simulink model "DynamicsAaa"  (R2017a)
(part 4 of 8)

v31 = 0.00359211102*c4*(- qd(3)*s3*(qd(1) + qd(2))) - 90*c4*(m6*(-c5*(- 295*c3^2*(qd(1) + qd(2))^2 + s2*(- 270*qd(1)^2) - 295*s3^2*(qd(1) + qd(2))^2) - s5*(c4*(+ c3*(c2*(- 270*qd(1)^2) - (qd(1) + qd(2))*(90*qd(1) + 90*qd(2)))) - s4*(- s3*(c2*(- 270*qd(1)^2) - (qd(1) + qd(2))*(90*qd(1) + 90*qd(2)))))) + m7*(c4*( - s3*(c2*(- 270*qd(1)^2) - (qd(1) + qd(2))*(90*qd(1) + 90*qd(2)))) + s4*( c3*(c2*(- 270*qd(1)^2) - (qd(1) + qd(2))*(90*qd(1) + 90*qd(2)))) + (-c5*(-qd(3) + qd(4)) - s5*(-c3*s4*(qd(1) + qd(2)) + c4*s3*(qd(1) + qd(2))))*(80*c5*(-qd(3) + qd(4)) + 80*s5*(-c3*s4*(qd(1) + qd(2)) + c4*s3*(qd(1) + qd(2)))) - (c5*(-c3*s4*(qd(1) + qd(2)) + c4*s3*(qd(1) + qd(2))) - s5*(-qd(3) + qd(4)))*(80*c5*(-c3*s4*(qd(1) + qd(2)) + c4*s3*(qd(1) + qd(2))) - 80*s5*(-qd(3) + qd(4))) - (-c6*(-c5*(-qd(3) + qd(4)) - s5*(-c3*s4*(qd(1) + qd(2)) + c4*s3*(qd(1) + qd(2)))) - s6*(c5*(-c3*s4*(qd(1) + qd(2)) + c4*s3*(qd(1) + qd(2))) - s5*(-qd(3) + qd(4))))*(80*c6*(-c5*(-qd(3) + qd(4)) - s5*(-c3*s4*(qd(1) + qd(2)) + c4*s3*(qd(1) + qd(2)))) + 80*s6*(c5*(-c3*s4*(qd(1) + qd(2)) + c4*s3*(qd(1) + qd(2))) - s5*(-qd(3) + qd(4)))) + (c6*(c5*(-c3*s4*(qd(1) + qd(2)) + c4*s3*(qd(1) + qd(2))) - s5*(-qd(3) + qd(4))) - s6*(-c5*(-qd(3) + qd(4)) - s5*(-c3*s4*(qd(1) + qd(2)) + c4*s3*(qd(1) + qd(2)))))*(80*c6*(c5*(-c3*s4*(qd(1) + qd(2)) + c4*s3*(qd(1) + qd(2))) - s5*(-qd(3) + qd(4))) - 80*s6*(-c5*(-qd(3) + qd(4)) - s5*(-c3*s4*(qd(1) + qd(2)) + c4*s3*(qd(1) + qd(2))))))) - 8.41256e-6*c4*(c3*qd(3)*(qd(1) + qd(2))) + c5*(-3.01352e-6*c6*(- qd(5)*(c5*(-c3*s4*(qd(1) + qd(2)) + c4*s3*(qd(1) + qd(2))) - s5*(-qd(3) + qd(4))) - s5*(c4*(c3*qd(3)*(qd(1) + qd(2))) + qd(4)*(-c3*c4*(qd(1) + qd(2)) - s3*s4*(qd(1) + qd(2))) - s4*( - qd(3)*s3*(qd(1) + qd(2))))) - 3.01352e-6*qd(6)*(c6*(c5*(-c3*s4*(qd(1) + qd(2)) + c4*s3*(qd(1) + qd(2))) - s5*(-qd(3) + qd(4))) - s6*(-c5*(-qd(3) + qd(4)) - s5*(-c3*s4*(qd(1) + qd(2)) + c4*s3*(qd(1) + qd(2))))) - 3.01352e-6*s6*(c5*(c4*(c3*qd(3)*(qd(1) + qd(2))) + qd(4)*(-c3*c4*(qd(1) + qd(2)) - s3*s4*(qd(1) + qd(2))) - s4*(- qd(3)*s3*(qd(1) + qd(2)))) + qd(5)*(-c5*(-qd(3) + qd(4)) - s5*(-c3*s4*(qd(1) + qd(2)) + c4*s3*(qd(1) + qd(2))))) + (6.20477e-6*c6*(c5*(-c3*s4*(qd(1) + qd(2)) + c4*s3*(qd(1) + qd(2))) - s5*(-qd(3) + qd(4))) - 6.20477e-6*s6*(-c5*(-qd(3) + qd(4)) - s5*(-c3*s4*(qd(1) + qd(2)) + c4*s3*(qd(1) + qd(2)))))*(c3*c4*(qd(1) + qd(2)) - qd(5) + qd(6) + s3*s4*(qd(1) + qd(2))) - (c6*(c5*(-c3*s4*(qd(1) + qd(2)) + c4*s3*(qd(1) + qd(2))) - s5*(-qd(3) + qd(4))) - s6*(-c5*(-qd(3) + qd(4)) - s5*(-c3*s4*(qd(1) + qd(2)) + c4*s3*(qd(1) + qd(2)))))*(3.29301e-6*c3*c4*(qd(1) + qd(2)) - 3.29301e-6*qd(5) + 3.29301e-6*qd(6) + 3.29301e-6*s3*s4*(qd(1) + qd(2)))) + 90*m5*(-c4*( - s3*(c2*(- 270*qd(1)^2) - (qd(1) + qd(2))*(90*qd(1) + 90*qd(2)))) + 295*c4*(c3*qd(3)*(qd(1) + qd(2))) + 295*qd(4)*(-c3*c4*(qd(1) + qd(2)) - s3*s4*(qd(1) + qd(2))) - s4*( c3*(c2*(- 270*qd(1)^2) - (qd(1) + qd(2))*(90*qd(1) + 90*qd(2)))) - 295*s4*(- qd(3)*s3*(qd(1) + qd(2))) + (-qd(3) + qd(4))*(295*c3*c4*(qd(1) + qd(2)) + 295*s3*s4*(qd(1) + qd(2)))) - 8.41256e-6*qd(4)*(-c3*c4*(qd(1) + qd(2)) - s3*s4*(qd(1) + qd(2))) + 0.00359211102*qd(4)*(-c3*s4*(qd(1) + qd(2)) + c4*s3*(qd(1) + qd(2))) + 8.41256e-6*s4*(- qd(3)*s3*(qd(1) + qd(2))) + 0.00359211102*s4*(c3*qd(3)*(qd(1) + qd(2))) - 90*s4*(c5*m7*(80*c6*(- qd(5)*(c5*(-c3*s4*(qd(1) + qd(2)) + c4*s3*(qd(1) + qd(2))) - s5*(-qd(3) + qd(4))) - s5*(c4*(c3*qd(3)*(qd(1) + qd(2))) + qd(4)*(-c3*c4*(qd(1) + qd(2)) - s3*s4*(qd(1) + qd(2))) - s4*(- qd(3)*s3*(qd(1) + qd(2))))) + c6*(c5*(c4*(c3*(c2*(- 270*qd(1)^2) - (qd(1) + qd(2))*(90*qd(1) + 90*qd(2)))) - s4*(- s3*(c2*(- 270*qd(1)^2) - (qd(1) + qd(2))*(90*qd(1) + 90*qd(2))))) + 80*qd(5)*(c5*(-c3*s4*(qd(1) + qd(2)) + c4*s3*(qd(1) + qd(2))) - s5*(-qd(3) + qd(4))) + 80*s5*(c4*(c3*qd(3)*(qd(1) + qd(2))) + qd(4)*(-c3*c4*(qd(1) + qd(2)) - s3*s4*(qd(1) + qd(2))) - s4*(- qd(3)*s3*(qd(1) + qd(2)))) - s5*(- 295*c3^2*(qd(1) + qd(2))^2 + s2*(- 270*qd(1)^2) - 295*s3^2*(qd(1) + qd(2))^2) - (80*c5*(-c3*s4*(qd(1) + qd(2)) + c4*s3*(qd(1) + qd(2))) - 80*s5*(-qd(3) + qd(4)))*(-c3*c4*(qd(1) + qd(2)) + qd(5) - s3*s4*(qd(1) + qd(2)))) + 80*qd(6)*(c6*(c5*(-c3*s4*(qd(1) + qd(2)) + c4*s3*(qd(1) + qd(2))) - s5*(-qd(3) + qd(4))) - s6*(-c5*(-qd(3) + qd(4)) - s5*(-c3*s4*(qd(1) + qd(2)) + c4*s3*(qd(1) + qd(2))))) + 80*s6*(c5*(c4*(c3*qd(3)*(qd(1) + qd(2))) + qd(4)*(-c3*c4*(qd(1) + qd(2)) - s3*s4*(qd(1) + qd(2))) - s4*(- qd(3)*s3*(qd(1) + qd(2)))) + qd(5)*(-c5*(-qd(3) + qd(4)) - s5*(-c3*s4*(qd(1) + qd(2)) + c4*s3*(qd(1) + qd(2))))) - s6*(80*c5*(c4*(c3*qd(3)*(qd(1) + qd(2))) + qd(4)*(-c3*c4*(qd(1) + qd(2)) - s3*s4*(qd(1) + qd(2))) - s4*(- qd(3)*s3*(qd(1) + qd(2)))) - c5*(- 295*c3^2*(qd(1) + qd(2))^2 + s2*(- 270*qd(1)^2) - 295*s3^2*(qd(1) + qd(2))^2) + 80*qd(5)*(-c5*(-qd(3) + qd(4)) - s5*(-c3*s4*(qd(1) + qd(2)) + c4*s3*(qd(1) + qd(2)))) - s5*(c4*(c3*(c2*(- 270*qd(1)^2) - (qd(1) + qd(2))*(90*qd(1) + 90*qd(2)))) - s4*(- s3*(c2*(- 270*qd(1)^2) - (qd(1) + qd(2))*(90*qd(1) + 90*qd(2))))) + (80*c5*(-qd(3) + qd(4)) + 80*s5*(-c3*s4*(qd(1) + qd(2)) + c4*s3*(qd(1) + qd(2))))*(-c3*c4*(qd(1) + qd(2)) + qd(5) - s3*s4*(qd(1) + qd(2)))) - (80*c6*(c5*(-c3*s4*(qd(1) + qd(2)) + c4*s3*(qd(1) + qd(2))) - s5*(-qd(3) + qd(4))) - 80*s6*(-c5*(-qd(3) + qd(4)) - s5*(-c3*s4*(qd(1) + qd(2)) + c4*s3*(qd(1) + qd(2)))))*(c3*c4*(qd(1) + qd(2)) - qd(5) + qd(6) + s3*s4*(qd(1) + qd(2)))) + m6*(c5*(c4*(c3*(c2*(- 270*qd(1)^2) - (qd(1) + qd(2))*(90*qd(1) + 90*qd(2)))) - s4*(- s3*(c2*(- 270*qd(1)^2) - (qd(1) + qd(2))*(90*qd(1) + 90*qd(2))))) - s5*( - 295*c3^2*(qd(1) + qd(2))^2 + s2*(- 270*qd(1)^2) - 295*s3^2*(qd(1) + qd(2))^2)) - m7*s5*(80*c6*(c5*(c4*(c3*qd(3)*(qd(1) + qd(2))) + qd(4)*(-c3*c4*(qd(1) + qd(2)) - s3*s4*(qd(1) + qd(2))) - s4*(- qd(3)*s3*(qd(1) + qd(2)))) + qd(5)*(-c5*(-qd(3) + qd(4)) - s5*(-c3*s4*(qd(1) + qd(2)) + c4*s3*(qd(1) + qd(2))))) - c6*(80*c5*(c4*(c3*qd(3)*(qd(1) + qd(2))) + qd(4)*(-c3*c4*(qd(1) + qd(2)) - s3*s4*(qd(1) + qd(2))) - s4*( - qd(3)*s3*(qd(1) + qd(2)))) - c5*( - 295*c3^2*(qd(1) + qd(2))^2 + s2*(- 270*qd(1)^2) - 295*s3^2*(qd(1) + qd(2))^2) + 80*qd(5)*(-c5*(-qd(3) + qd(4)) - s5*(-c3*s4*(qd(1) + qd(2)) + c4*s3*(qd(1) + qd(2)))) - s5*(c4*(c3*(c2*(- 270*qd(1)^2) - (qd(1) + qd(2))*(90*qd(1) + 90*qd(2)))) - s4*(- s3*(c2*(- 270*qd(1)^2) - (qd(1) + qd(2))*(90*qd(1) + 90*qd(2))))) + (80*c5*(-qd(3) + qd(4)) + 80*s5*(-c3*s4*(qd(1) + qd(2)) + c4*s3*(qd(1) + qd(2))))*(-c3*c4*(qd(1) + qd(2)) + qd(5) - s3*s4*(qd(1) + qd(2)))) + 80*qd(6)*(-c6*(-c5*(-qd(3) + qd(4)) - s5*(-c3*s4*(qd(1) + qd(2)) + c4*s3*(qd(1) + qd(2)))) - s6*(c5*(-c3*s4*(qd(1) + qd(2)) + c4*s3*(qd(1) + qd(2))) - s5*(-qd(3) + qd(4)))) - 80*s6*(- qd(5)*(c5*(-c3*s4*(qd(1) + qd(2)) + c4*s3*(qd(1) + qd(2))) - s5*(-qd(3) + qd(4))) - s5*(c4*(c3*qd(3)*(qd(1) + qd(2))) + qd(4)*(-c3*c4*(qd(1) + qd(2)) - s3*s4*(qd(1) + qd(2))) - s4*(- qd(3)*s3*(qd(1) + qd(2))))) - s6*(c5*(c4*(c3*(c2*(- 270*qd(1)^2) - (qd(1) + qd(2))*(90*qd(1) + 90*qd(2)))) - s4*( - s3*(c2*(- 270*qd(1)^2) - (qd(1) + qd(2))*(90*qd(1) + 90*qd(2))))) + 80*qd(5)*(c5*(-c3*s4*(qd(1) + qd(2)) + c4*s3*(qd(1) + qd(2))) - s5*(-qd(3) + qd(4))) + 80*s5*(c4*(c3*qd(3)*(qd(1) + qd(2))) + qd(4)*(-c3*c4*(qd(1) + qd(2)) - s3*s4*(qd(1) + qd(2))) - s4*(- qd(3)*s3*(qd(1) + qd(2)))) - s5*(- 295*c3^2*(qd(1) + qd(2))^2 + s2*(- 270*qd(1)^2) - 295*s3^2*(qd(1) + qd(2))^2) - (80*c5*(-c3*s4*(qd(1) + qd(2)) + c4*s3*(qd(1) + qd(2))) - 80*s5*(-qd(3) + qd(4)))*(-c3*c4*(qd(1) + qd(2)) + qd(5) - s3*s4*(qd(1) + qd(2)))) + (80*c6*(-c5*(-qd(3) + qd(4)) - s5*(-c3*s4*(qd(1) + qd(2)) + c4*s3*(qd(1) + qd(2)))) + 80*s6*(c5*(-c3*s4*(qd(1) + qd(2)) + c4*s3*(qd(1) + qd(2))) - s5*(-qd(3) + qd(4))))*(c3*c4*(qd(1) + qd(2)) - qd(5) + qd(6) + s3*s4*(qd(1) + qd(2))))) + s5*(6.20477e-6*c6*(c5*(c4*(c3*qd(3)*(qd(1) + qd(2))) + qd(4)*(-c3*c4*(qd(1) + qd(2)) - s3*s4*(qd(1) + qd(2))) - s4*(- qd(3)*s3*(qd(1) + qd(2)))) + qd(5)*(-c5*(-qd(3) + qd(4)) - s5*(-c3*s4*(qd(1) + qd(2)) + c4*s3*(qd(1) + qd(2))))) + 6.20477e-6*qd(6)*(-c6*(-c5*(-qd(3) + qd(4)) - s5*(-c3*s4*(qd(1) + qd(2)) + c4*s3*(qd(1) + qd(2)))) - s6*(c5*(-c3*s4*(qd(1) + qd(2)) + c4*s3*(qd(1) + qd(2))) - s5*(-qd(3) + qd(4)))) - 6.20477e-6*s6*(- qd(5)*(c5*(-c3*s4*(qd(1) + qd(2)) + c4*s3*(qd(1) + qd(2))) - s5*(-qd(3) + qd(4))) - s5*(c4*(c3*qd(3)*(qd(1) + qd(2))) + qd(4)*(-c3*c4*(qd(1) + qd(2)) - s3*s4*(qd(1) + qd(2))) - s4*(- qd(3)*s3*(qd(1) + qd(2))))) + (-c6*(-c5*(-qd(3) + qd(4)) - s5*(-c3*s4*(qd(1) + qd(2)) + c4*s3*(qd(1) + qd(2)))) - s6*(c5*(-c3*s4*(qd(1) + qd(2)) + c4*s3*(qd(1) + qd(2))) - s5*(-qd(3) + qd(4))))*(3.29301e-6*c3*c4*(qd(1) + qd(2)) - 3.29301e-6*qd(5) + 3.29301e-6*qd(6) + 3.29301e-6*s3*s4*(qd(1) + qd(2))) - (-3.01352e-6*c6*(-c5*(-qd(3) + qd(4)) - s5*(-c3*s4*(qd(1) + qd(2)) + c4*s3*(qd(1) + qd(2)))) - 3.01352e-6*s6*(c5*(-c3*s4*(qd(1) + qd(2)) + c4*s3*(qd(1) + qd(2))) - s5*(-qd(3) + qd(4))))*(c3*c4*(qd(1) + qd(2)) - qd(5) + qd(6) + s3*s4*(qd(1) + qd(2)))) + (-c5*(-qd(3) + qd(4)) - s5*(-c3*s4*(qd(1) + qd(2)) + c4*s3*(qd(1) + qd(2))))*(0.000409305*c5*(-qd(3) + qd(4)) + 0.00151607*c5*(-c3*s4*(qd(1) + qd(2)) + c4*s3*(qd(1) + qd(2))) - 0.00151607*s5*(-qd(3) + qd(4)) + 0.000409305*s5*(-c3*s4*(qd(1) + qd(2)) + c4*s3*(qd(1) + qd(2)))) - (c5*(-c3*s4*(qd(1) + qd(2)) + c4*s3*(qd(1) + qd(2))) - s5*(-qd(3) + qd(4)))*(-0.00355535*c5*(-qd(3) + qd(4)) - 0.000409305*c5*(-c3*s4*(qd(1) + qd(2)) + c4*s3*(qd(1) + qd(2))) + 0.000409305*s5*(-qd(3) + qd(4)) - 0.00355535*s5*(-c3*s4*(qd(1) + qd(2)) + c4*s3*(qd(1) + qd(2)))) - (-c3*c4*(qd(1) + qd(2)) - s3*s4*(qd(1) + qd(2)))*(0.00163355*c3*c4*(qd(1) + qd(2)) - 0.00950111*c3*s4*(qd(1) + qd(2)) + 0.00950111*c4*s3*(qd(1) + qd(2)) + 8.41256e-6*qd(3) - 8.41256e-6*qd(4) + 0.00163355*s3*s4*(qd(1) + qd(2))) + (-c3*s4*(qd(1) + qd(2)) + c4*s3*(qd(1) + qd(2)))*(-0.020170031*c3*c4*(qd(1) + qd(2)) + 0.00163355*c3*s4*(qd(1) + qd(2)) - 0.00163355*c4*s3*(qd(1) + qd(2)) + 2.69102e-6*qd(3) - 2.69102e-6*qd(4) - 0.020170031*s3*s4*(qd(1) + qd(2)));

v41 = -0.00358942*c4*( - qd(3)*s3*(qd(1) + qd(2))) - c5*(-3.01352e-6*c6*(- qd(5)*(c5*(-c3*s4*(qd(1) + qd(2)) + c4*s3*(qd(1) + qd(2))) - s5*(-qd(3) + qd(4))) - s5*(c4*(c3*qd(3)*(qd(1) + qd(2))) + qd(4)*(-c3*c4*(qd(1) + qd(2)) - s3*s4*(qd(1) + qd(2))) - s4*(- qd(3)*s3*(qd(1) + qd(2))))) - 3.01352e-6*qd(6)*(c6*(c5*(-c3*s4*(qd(1) + qd(2)) + c4*s3*(qd(1) + qd(2))) - s5*(-qd(3) + qd(4))) - s6*(-c5*(-qd(3) + qd(4)) - s5*(-c3*s4*(qd(1) + qd(2)) + c4*s3*(qd(1) + qd(2))))) - 3.01352e-6*s6*(c5*(c4*(c3*qd(3)*(qd(1) + qd(2))) + qd(4)*(-c3*c4*(qd(1) + qd(2)) - s3*s4*(qd(1) + qd(2))) - s4*(- qd(3)*s3*(qd(1) + qd(2)))) + qd(5)*(-c5*(-qd(3) + qd(4)) - s5*(-c3*s4*(qd(1) + qd(2)) + c4*s3*(qd(1) + qd(2))))) + (6.20477e-6*c6*(c5*(-c3*s4*(qd(1) + qd(2)) + c4*s3*(qd(1) + qd(2))) - s5*(-qd(3) + qd(4))) - 6.20477e-6*s6*(-c5*(-qd(3) + qd(4)) - s5*(-c3*s4*(qd(1) + qd(2)) + c4*s3*(qd(1) + qd(2)))))*(c3*c4*(qd(1) + qd(2)) - qd(5) + qd(6) + s3*s4*(qd(1) + qd(2))) - (c6*(c5*(-c3*s4*(qd(1) + qd(2)) + c4*s3*(qd(1) + qd(2))) - s5*(-qd(3) + qd(4))) - s6*(-c5*(-qd(3) + qd(4)) - s5*(-c3*s4*(qd(1) + qd(2)) + c4*s3*(qd(1) + qd(2)))))*(3.29301e-6*c3*c4*(qd(1) + qd(2)) - 3.29301e-6*qd(5) + 3.29301e-6*qd(6) + 3.29301e-6*s3*s4*(qd(1) + qd(2)))) - 0.00358942*qd(4)*(-c3*s4*(qd(1) + qd(2)) + c4*s3*(qd(1) + qd(2))) - 0.00358942*s4*(c3*qd(3)*(qd(1) + qd(2))) - s5*(6.20477e-6*c6*(c5*(c4*(c3*qd(3)*(qd(1) + qd(2))) + qd(4)*(-c3*c4*(qd(1) + qd(2)) - s3*s4*(qd(1) + qd(2))) - s4*( - qd(3)*s3*(qd(1) + qd(2)))) + qd(5)*(-c5*(-qd(3) + qd(4)) - s5*(-c3*s4*(qd(1) + qd(2)) + c4*s3*(qd(1) + qd(2))))) + 6.20477e-6*qd(6)*(-c6*(-c5*(-qd(3) + qd(4)) - s5*(-c3*s4*(qd(1) + qd(2)) + c4*s3*(qd(1) + qd(2)))) - s6*(c5*(-c3*s4*(qd(1) + qd(2)) + c4*s3*(qd(1) + qd(2))) - s5*(-qd(3) + qd(4)))) - 6.20477e-6*s6*(- qd(5)*(c5*(-c3*s4*(qd(1) + qd(2)) + c4*s3*(qd(1) + qd(2))) - s5*(-qd(3) + qd(4))) - s5*(c4*(c3*qd(3)*(qd(1) + qd(2))) + qd(4)*(-c3*c4*(qd(1) + qd(2)) - s3*s4*(qd(1) + qd(2))) - s4*(- qd(3)*s3*(qd(1) + qd(2))))) + (-c6*(-c5*(-qd(3) + qd(4)) - s5*(-c3*s4*(qd(1) + qd(2)) + c4*s3*(qd(1) + qd(2)))) - s6*(c5*(-c3*s4*(qd(1) + qd(2)) + c4*s3*(qd(1) + qd(2))) - s5*(-qd(3) + qd(4))))*(3.29301e-6*c3*c4*(qd(1) + qd(2)) - 3.29301e-6*qd(5) + 3.29301e-6*qd(6) + 3.29301e-6*s3*s4*(qd(1) + qd(2))) - (-3.01352e-6*c6*(-c5*(-qd(3) + qd(4)) - s5*(-c3*s4*(qd(1) + qd(2)) + c4*s3*(qd(1) + qd(2)))) - 3.01352e-6*s6*(c5*(-c3*s4*(qd(1) + qd(2)) + c4*s3*(qd(1) + qd(2))) - s5*(-qd(3) + qd(4))))*(c3*c4*(qd(1) + qd(2)) - qd(5) + qd(6) + s3*s4*(qd(1) + qd(2)))) - (-c5*(-qd(3) + qd(4)) - s5*(-c3*s4*(qd(1) + qd(2)) + c4*s3*(qd(1) + qd(2))))*(0.000409305*c5*(-qd(3) + qd(4)) + 0.00151607*c5*(-c3*s4*(qd(1) + qd(2)) + c4*s3*(qd(1) + qd(2))) - 0.00151607*s5*(-qd(3) + qd(4)) + 0.000409305*s5*(-c3*s4*(qd(1) + qd(2)) + c4*s3*(qd(1) + qd(2)))) + (c5*(-c3*s4*(qd(1) + qd(2)) + c4*s3*(qd(1) + qd(2))) - s5*(-qd(3) + qd(4)))*(-0.00355535*c5*(-qd(3) + qd(4)) - 0.000409305*c5*(-c3*s4*(qd(1) + qd(2)) + c4*s3*(qd(1) + qd(2))) + 0.000409305*s5*(-qd(3) + qd(4)) - 0.00355535*s5*(-c3*s4*(qd(1) + qd(2)) + c4*s3*(qd(1) + qd(2))));

v51 = 3.29301e-6*c4*(- qd(3)*s3*(qd(1) + qd(2))) + 3.29301e-6*qd(4)*(-c3*s4*(qd(1) + qd(2)) + c4*s3*(qd(1) + qd(2))) + 3.29301e-6*s4*(c3*qd(3)*(qd(1) + qd(2))) - (-c6*(-c5*(-qd(3) + qd(4)) - s5*(-c3*s4*(qd(1) + qd(2)) + c4*s3*(qd(1) + qd(2)))) - s6*(c5*(-c3*s4*(qd(1) + qd(2)) + c4*s3*(qd(1) + qd(2))) - s5*(-qd(3) + qd(4))))*(6.20477e-6*c6*(c5*(-c3*s4*(qd(1) + qd(2)) + c4*s3*(qd(1) + qd(2))) - s5*(-qd(3) + qd(4))) - 6.20477e-6*s6*(-c5*(-qd(3) + qd(4)) - s5*(-c3*s4*(qd(1) + qd(2)) + c4*s3*(qd(1) + qd(2))))) + (-3.01352e-6*c6*(-c5*(-qd(3) + qd(4)) - s5*(-c3*s4*(qd(1) + qd(2)) + c4*s3*(qd(1) + qd(2)))) - 3.01352e-6*s6*(c5*(-c3*s4*(qd(1) + qd(2)) + c4*s3*(qd(1) + qd(2))) - s5*(-qd(3) + qd(4))))*(c6*(c5*(-c3*s4*(qd(1) + qd(2)) + c4*s3*(qd(1) + qd(2))) - s5*(-qd(3) + qd(4))) - s6*(-c5*(-qd(3) + qd(4)) - s5*(-c3*s4*(qd(1) + qd(2)) + c4*s3*(qd(1) + qd(2)))));

v61 = 0;

V = [v11 ; v21 ; v31 ; v41 ; v51 ; v61];
%% matrix G



% g1 = diff(tau1,g)*g ;
% g2 = diff(tau2,g)*g ;
% g3 = diff(tau3,g)*g ;
% g4 = diff(tau4,g)*g ;
% g5 = diff(tau5,g)*g ;
% g6 = diff(tau6,g)*g ;

g1 = g*(335*c2*(c3*(m5*(s3*s4*(c1*s2 + c2*s1) + c3*c4*(c1*s2 + c2*s1)) - s4*(m7*(c3*s4*(c1*s2 + c2*s1) - c4*s3*(c1*s2 + c2*s1)) - m6*(s5*(s3*s4*(c1*s2 + c2*s1) + c3*c4*(c1*s2 + c2*s1)) - c5*(c1*c2 - s1*s2))) + c4*(m6*(c5*(s3*s4*(c1*s2 + c2*s1) + c3*c4*(c1*s2 + c2*s1)) + s5*(c1*c2 - s1*s2)) + c5*m7*(c6*(c5*(s3*s4*(c1*s2 + c2*s1) + c3*c4*(c1*s2 + c2*s1)) + s5*(c1*c2 - s1*s2)) + s6*(s5*(s3*s4*(c1*s2 + c2*s1) + c3*c4*(c1*s2 + c2*s1)) - c5*(c1*c2 - s1*s2))) - m7*s5*(c6*(s5*(s3*s4*(c1*s2 + c2*s1) + c3*c4*(c1*s2 + c2*s1)) - c5*(c1*c2 - s1*s2)) - s6*(c5*(s3*s4*(c1*s2 + c2*s1) + c3*c4*(c1*s2 + c2*s1)) + s5*(c1*c2 - s1*s2))))) + s3*(m5*(c3*s4*(c1*s2 + c2*s1) - c4*s3*(c1*s2 + c2*s1)) + c4*(m7*(c3*s4*(c1*s2 + c2*s1) - c4*s3*(c1*s2 + c2*s1)) - m6*(s5*(s3*s4*(c1*s2 + c2*s1) + c3*c4*(c1*s2 + c2*s1)) - c5*(c1*c2 - s1*s2))) + s4*(m6*(c5*(s3*s4*(c1*s2 + c2*s1) + c3*c4*(c1*s2 + c2*s1)) + s5*(c1*c2 - s1*s2)) + c5*m7*(c6*(c5*(s3*s4*(c1*s2 + c2*s1) + c3*c4*(c1*s2 + c2*s1)) + s5*(c1*c2 - s1*s2)) + s6*(s5*(s3*s4*(c1*s2 + c2*s1) + c3*c4*(c1*s2 + c2*s1)) - c5*(c1*c2 - s1*s2))) - m7*s5*(c6*(s5*(s3*s4*(c1*s2 + c2*s1) + c3*c4*(c1*s2 + c2*s1)) - c5*(c1*c2 - s1*s2)) - s6*(c5*(s3*s4*(c1*s2 + c2*s1) + c3*c4*(c1*s2 + c2*s1)) + s5*(c1*c2 - s1*s2))))) + c3*m4*(c1*s2 + c2*s1)) - 75*c2*(m6*(c3*s4*(c1*s2 + c2*s1) - c4*s3*(c1*s2 + c2*s1)) - m5*(c1*c2 - s1*s2) - m4*s3*(c1*s2 + c2*s1) + c5*m7*(c6*(s5*(s3*s4*(c1*s2 + c2*s1) + c3*c4*(c1*s2 + c2*s1)) - c5*(c1*c2 - s1*s2)) - s6*(c5*(s3*s4*(c1*s2 + c2*s1) + c3*c4*(c1*s2 + c2*s1)) + s5*(c1*c2 - s1*s2))) + m7*s5*(c6*(c5*(s3*s4*(c1*s2 + c2*s1) + c3*c4*(c1*s2 + c2*s1)) + s5*(c1*c2 - s1*s2)) + s6*(s5*(s3*s4*(c1*s2 + c2*s1) + c3*c4*(c1*s2 + c2*s1)) - c5*(c1*c2 - s1*s2)))) + c3*(90*m6*(c3*s4*(c1*s2 + c2*s1) - c4*s3*(c1*s2 + c2*s1)) + s4*(295*m7*(c3*s4*(c1*s2 + c2*s1) - c4*s3*(c1*s2 + c2*s1)) - 295*m6*(s5*(s3*s4*(c1*s2 + c2*s1) + c3*c4*(c1*s2 + c2*s1)) - c5*(c1*c2 - s1*s2))) - 90*m5*(c1*c2 - s1*s2) - c4*(295*m6*(c5*(s3*s4*(c1*s2 + c2*s1) + c3*c4*(c1*s2 + c2*s1)) + s5*(c1*c2 - s1*s2)) + 295*c5*m7*(c6*(c5*(s3*s4*(c1*s2 + c2*s1) + c3*c4*(c1*s2 + c2*s1)) + s5*(c1*c2 - s1*s2)) + s6*(s5*(s3*s4*(c1*s2 + c2*s1) + c3*c4*(c1*s2 + c2*s1)) - c5*(c1*c2 - s1*s2))) - 295*m7*s5*(c6*(s5*(s3*s4*(c1*s2 + c2*s1) + c3*c4*(c1*s2 + c2*s1)) - c5*(c1*c2 - s1*s2)) - s6*(c5*(s3*s4*(c1*s2 + c2*s1) + c3*c4*(c1*s2 + c2*s1)) + s5*(c1*c2 - s1*s2)))) + 90*c5*m7*(c6*(s5*(s3*s4*(c1*s2 + c2*s1) + c3*c4*(c1*s2 + c2*s1)) - c5*(c1*c2 - s1*s2)) - s6*(c5*(s3*s4*(c1*s2 + c2*s1) + c3*c4*(c1*s2 + c2*s1)) + s5*(c1*c2 - s1*s2))) + 90*m7*s5*(c6*(c5*(s3*s4*(c1*s2 + c2*s1) + c3*c4*(c1*s2 + c2*s1)) + s5*(c1*c2 - s1*s2)) + s6*(s5*(s3*s4*(c1*s2 + c2*s1) + c3*c4*(c1*s2 + c2*s1)) - c5*(c1*c2 - s1*s2)))) - 270*c5*m7*(75*s2*(c3*(m5*(s3*s4*(c1*s2 + c2*s1) + c3*c4*(c1*s2 + c2*s1)) - s4*(m7*(c3*s4*(c1*s2 + c2*s1) - c4*s3*(c1*s2 + c2*s1)) - m6*(s5*(s3*s4*(c1*s2 + c2*s1) + c3*c4*(c1*s2 + c2*s1)) - c5*(c1*c2 - s1*s2))) + c4*(m6*(c5*(s3*s4*(c1*s2 + c2*s1) + c3*c4*(c1*s2 + c2*s1)) + s5*(c1*c2 - s1*s2)) + c5*m7*(c6*(c5*(s3*s4*(c1*s2 + c2*s1) + c3*c4*(c1*s2 + c2*s1)) + s5*(c1*c2 - s1*s2)) + s6*(s5*(s3*s4*(c1*s2 + c2*s1) + c3*c4*(c1*s2 + c2*s1)) - c5*(c1*c2 - s1*s2))) - m7*s5*(c6*(s5*(s3*s4*(c1*s2 + c2*s1) + c3*c4*(c1*s2 + c2*s1)) - c5*(c1*c2 - s1*s2)) - s6*(c5*(s3*s4*(c1*s2 + c2*s1) + c3*c4*(c1*s2 + c2*s1)) + s5*(c1*c2 - s1*s2))))) + s3*(m5*(c3*s4*(c1*s2 + c2*s1) - c4*s3*(c1*s2 + c2*s1)) + c4*(m7*(c3*s4*(c1*s2 + c2*s1) - c4*s3*(c1*s2 + c2*s1)) - m6*(s5*(s3*s4*(c1*s2 + c2*s1) + c3*c4*(c1*s2 + c2*s1)) - c5*(c1*c2 - s1*s2))) + s4*(m6*(c5*(s3*s4*(c1*s2 + c2*s1) + c3*c4*(c1*s2 + c2*s1)) + s5*(c1*c2 - s1*s2)) + c5*m7*(c6*(c5*(s3*s4*(c1*s2 + c2*s1) + c3*c4*(c1*s2 + c2*s1)) + s5*(c1*c2 - s1*s2)) + s6*(s5*(s3*s4*(c1*s2 + c2*s1) + c3*c4*(c1*s2 + c2*s1)) - c5*(c1*c2 - s1*s2))) - m7*s5*(c6*(s5*(s3*s4*(c1*s2 + c2*s1) + c3*c4*(c1*s2 + c2*s1)) - c5*(c1*c2 - s1*s2)) - s6*(c5*(s3*s4*(c1*s2 + c2*s1) + c3*c4*(c1*s2 + c2*s1)) + s5*(c1*c2 - s1*s2))))) + c3*m4*(c1*s2 + c2*s1)) + 270*m6*(c3*s4*(c1*s2 + c2*s1) - c4*s3*(c1*s2 + c2*s1)) + s3*(c4*(295*m7*(c3*s4*(c1*s2 + c2*s1) - c4*s3*(c1*s2 + c2*s1)) - 295*m6*(s5*(s3*s4*(c1*s2 + c2*s1) + c3*c4*(c1*s2 + c2*s1)) - c5*(c1*c2 - s1*s2))) + s4*(295*m6*(c5*(s3*s4*(c1*s2 + c2*s1) + c3*c4*(c1*s2 + c2*s1)) + s5*(c1*c2 - s1*s2)) + 295*c5*m7*(c6*(c5*(s3*s4*(c1*s2 + c2*s1) + c3*c4*(c1*s2 + c2*s1)) + s5*(c1*c2 - s1*s2)) + s6*(s5*(s3*s4*(c1*s2 + c2*s1) + c3*c4*(c1*s2 + c2*s1)) - c5*(c1*c2 - s1*s2))) - 295*m7*s5*(c6*(s5*(s3*s4*(c1*s2 + c2*s1) + c3*c4*(c1*s2 + c2*s1)) - c5*(c1*c2 - s1*s2)) - s6*(c5*(s3*s4*(c1*s2 + c2*s1) + c3*c4*(c1*s2 + c2*s1)) + s5*(c1*c2 - s1*s2))))) - c6*(c5*(c1*c2 + s5*(s3*s4*(c1*s2 + c2*s1) + c3*c4*(c1*s2 + c2*s1)) + 295*c3^2*s1*s2) - s6*(c5*(s3*s4*(c1*s2 + c2*s1) + c3*c4*(c1*s2 + c2*s1)) + s5*(c1*c2 - s1*s2))) - 335*m3*(c1*s2 + c2*s1) + 75*m3*(c1*c2 - s1*s2) - 270*m5*(c1*c2 - s1*s2) + 335*s2*(m6*(c3*s4*(c1*s2 + c2*s1) - c4*s3*(c1*s2 + c2*s1)) - m5*(c1*c2 - s1*s2) - m4*s3*(c1*s2 + c2*s1) + c5*m7*(c6*(s5*(s3*s4*(c1*s2 + c2*s1) + c3*c4*(c1*s2 + c2*s1)) - c5*(c1*c2 - s1*s2)) - s6*(c5*(s3*s4*(c1*s2 + c2*s1) + c3*c4*(c1*s2 + c2*s1)) + s5*(c1*c2 - s1*s2))) + m7*s5*(c6*(c5*(s3*s4*(c1*s2 + c2*s1) + c3*c4*(c1*s2 + c2*s1)) + s5*(c1*c2 - s1*s2)) + s6*(s5*(s3*s4*(c1*s2 + c2*s1) + c3*c4*(c1*s2 + c2*s1)) - c5*(c1*c2 - s1*s2)))) - 270*m4*s3*(c1*s2 + c2*s1) + 270*m7*s5*(c6*(c5*(s3*s4*(c1*s2 + c2*s1) + c3*c4*(c1*s2 + c2*s1)) + s5*(c1*c2 - s1*s2)) + s6*(s5*(s3*s4*(c1*s2 + c2*s1) + c3*c4*(c1*s2 + c2*s1)) - c5*(c1*c2 - s1*s2)))));
g2 = -c3*g*(270*m6*(c3*s4*(c1*s2 + c2*s1) - c4*s3*(c1*s2 + c2*s1)) + s3*(c4*(295*m7*(c3*s4*(c1*s2 + c2*s1) - c4*s3*(c1*s2 + c2*s1)) - 295*m6*(s5*(s3*s4*(c1*s2 + c2*s1) + c3*c4*(c1*s2 + c2*s1)) - c5*(c1*c2 - s1*s2))) - 295*c5*m7*s4*(s6*(c5*(c1*c2 - s1*s2) - s5*(c3*c4*(c1*s2 + c2*s1) + c2*s3*s4*(s1 + c1*s2))) - c6*(c5*(s3*s4*(c1*s2 + c2*s1) + c3*c4*(c1*s2 + c2*s1)) + s5*(c1*c2 - s1*s2)) + 295*m6*(c5*(s3*s4*(c1*s2 + c2*s1) + c3*c4*(c1*s2 + c2*s1)) + s5*(c1*c2 - s1*s2)) - 295*m7*s5*(c6*(s5*(s3*s4*(c1*s2 + c2*s1) + c3*c4*(c1*s2 + c2*s1)) - c5*(c1*c2 - s1*s2)) - s6*(c5*(s3*s4*(c1*s2 + c2*s1) + c3*c4*(c1*s2 + c2*s1)) + s5*(c1*c2 - s1*s2))))) - 270*m5*(c1*c2 - s1*s2) + c4*(90*m6*(c3*s4*(c1*s2 + c2*s1) - c4*s3*(c1*s2 + c2*s1)) + s4*(295*m7*(c3*s4*(c1*s2 + c2*s1) - c4*s3*(c1*s2 + c2*s1)) - 295*m6*(s5*(s3*s4*(c1*s2 + c2*s1) + c3*c4*(c1*s2 + c2*s1)) - c5*(c1*c2 - s1*s2))) + 295*m6*(c5*(s3*s4*(c1*s2 + c2*s1) + c3*c4*(c1*s2 + c2*s1)) + s5*(c1*c2 - s1*s2) + 295*m7*s5*(c6*(s5*(s3*s4*(c1*s2 + c2*s1) + c3*c4*(c1*s2 + c2*s1)) - c5*(c1*c2 - s1*s2)) - s6*(c5*(s3*s4*(c1*s2 + c2*s1) + c3*c4*(c1*s2 + c2*s1)) + s5*(c1*c2 - s1*s2)))) - 90*m5*(c1*c2 - s1*s2) + 295*c5*m7*(c6*(c5*(s3*s4*(c1*s2 + c2*s1) + c3*c4*(c1*s2 + c2*s1)) + s5*(c1*c2 - s1*s2)) + s6*(s5*(s3*s4*(c1*s2 + c2*s1) + c3*c4*(c1*s2 + c2*s1)) - c5*(c1*c2 - s1*s2))) + 90*c5*m7*(c6*(s5*(s3*s4*(c1*s2 + c2*s1) + c3*c4*(c1*s2 + c2*s1)) - c5*(c1*c2 - s1*s2)) - s6*(c5*(s3*s4*(c1*s2 + c2*s1) + c3*c4*(c1*s2 + c2*s1)) + s5*(c1*c2 - s1*s2))) + 90*m7*s5*(c6*(c5*(s3*s4*(c1*s2 + c2*s1) + c3*c4*(c1*s2 + c2*s1)) + s5*(c1*c2 - s1*s2)) + s6*(s5*(s3*s4*(c1*s2 + c2*s1) + c3*c4*(c1*s2 + c2*s1)) - c5*(c1*c2 - s1*s2)))) - 270*m4*s3*(c1*s2 + c2*s1) + 270*c5*m7*(c6*(s5*(s3*s4*(c1*s2 + c2*s1) + c3*c4*(c1*s2 + c2*s1)) - c5*(c1*c2 - s1*s2)) - s6*(c5*(s3*s4*(c1*s2 + c2*s1) + c3*c4*(c1*s2 + c2*s1)) + s5*(c1*c2 - s1*s2))) + 270*m7*s5*(c6*(c5*(s3*s4*(c1*s2 + c2*s1) + c3*c4*(c1*s2 + c2*s1)) + s5*(c1*c2 - s1*s2)) + s6*(s5*(s3*s4*(c1*s2 + c2*s1) + c3*c4*(c1*s2 + c2*s1)) - c5*(c1*c2 - s1*s2))));
g3 = g*(90*m5*(c3*s4*(c1*s2 + c2*s1) - c4*s3*(c1*s2 + c2*s1)) + 90*c4*(m7*(c3*s4*(c1*s2 + c2*s1) - c4*s3*(c1*s2 + c2*s1)) - m6*(s5*(s3*s4*(c1*s2 + c2*s1) + c3*c4*(c1*s2 + c2*s1)) - c5*(c1*c2 - s1*s2))) + 90*s4*(m6*(c5*(s3*s4*(c1*s2 + c2*s1) + c3*c4*(c1*s2 + c2*s1)) + s5*(c1*c2 - s1*s2)) + c5*m7*(c6*(c5*(s3*s4*(c1*s2 + c2*s1) + c3*c4*(c1*s2 + c2*s1)) + s5*(c1*c2 - s1*s2)) + s6*(s5*(s3*s4*(c1*s2 + c2*s1) + c3*c4*(c1*s2 + c2*s1)) - c5*(c1*c2 - s1*s2))) - m7*s5*(c6*(s5*(s3*s4*(c1*s2 + c2*s1) + c3*c4*(c1*s2 + c2*s1)) - c5*(c1*c2 - s1*s2)) - s6*(c5*(s3*s4*(c1*s2 + c2*s1) + c3*c4*(c1*s2 + c2*s1)) + s5*(c1*c2 - s1*s2)))))
g4 = 0;
g5 = 0;
g6 = 0;

G = [g1 ; g2 ; g3 ; g4 ; g5 ; g6] ;
%% out put

a = q_des_ddot - Kp*(q - q_des) - Kd*(qd - q_des_dot);
torque = M*a + V + G;
